simulink library "allActuatorPlant_cl"  (R2018b)
settings: Solver=VariableStepAuto  StartTime=0.0  StopTime=10.0  RelTol=1e-3
values from neighbouring files (symbols this model uses):
  unstretched_l = unstretched_l - ini_elongation - added_elongation    [ayazParams_init.m]    (also in multinode_wing_tail.m)
  X0 = cat(1,ini_Rcm_o,ini_O_Vcm_o,ini_euler_ang,ini_OwB,ini_platform_ang,ini_platform_vel,     ini_R1i_o,ini_R2i_o,ini_R3i_o,ini_O_V1i_o,ini_O_V2i_o,ini_O_V3i_o)    [ayazParams_init.m]    (also in multinode_wing_tail.m)
settings Model: Creator=mcobb  LastModifiedBy=embeato2

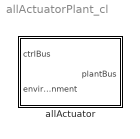
== system allActuatorPlant_cl ==
  allActuator : Subsystem

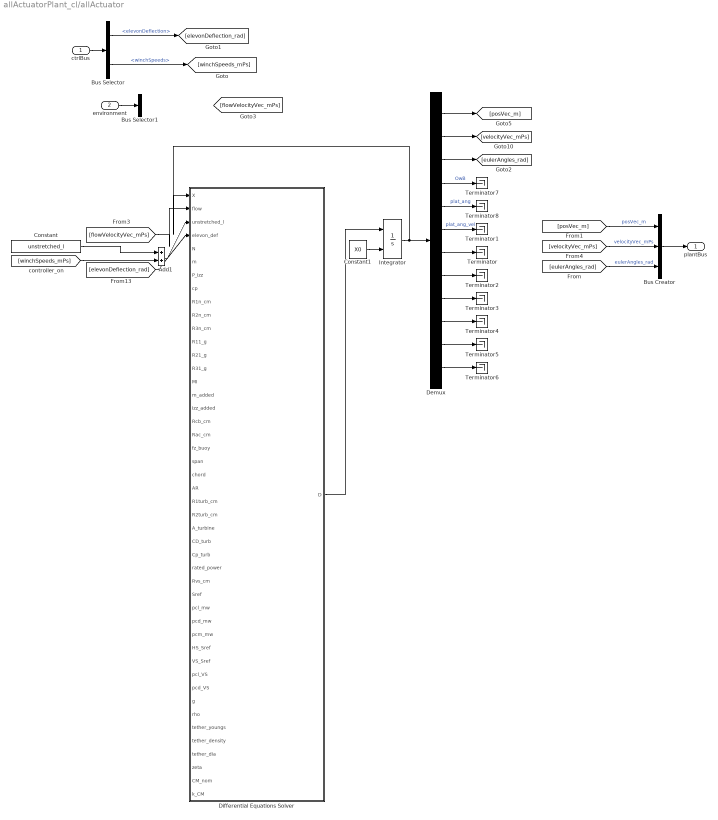
== system allActuatorPlant_cl/allActuator ==
  ctrlBus : Inport  OutDataTypeStr=Bus: ctrlBus
  environment : Inport  Port=2  OutDataTypeStr=Bus: envBus
  Add1 : Sum
  Bus Creator : BusCreator  Inputs=3  OutDataTypeStr=Bus: plantBus
  Bus Selector : BusSelector  OutputSignals=elevonDeflection,winchSpeeds
  Bus Selector1 : BusSelector  OutputSignals=windSpeed,windDir
  Constant : Constant  Value=unstretched_l
  Constant1 : Constant  Value=X0
  Demux : Demux  Outputs=[3,3,3,3,1,1,-1,-1,-1,-1,-1,-1]
  Differential Equations Solver : MATLAB Function  TreatAsAtomicUnit=on
  Integrator : Integrator  InitialConditionSource=external  InitialCondition=X0
  Terminator{,1..8} (9 alike) : Terminator
  plantBus : Outport  OutDataTypeStr=Bus: plantBus
  wires:
  Demux/3 -> [eulerAngles_rad]
  Integrator/1 -> Differential Equations Solver/1(X), Demux/1
  Demux/6 -> Terminator1/1  "plat_ang_vel"
  Constant/1 -> Add1/1
  Demux/7 -> Terminator/1
  Add1/1 -> Differential Equations Solver/3(unstretched_l)
  Differential Equations Solver/1(D) -> Integrator/1
  Demux/10 -> Terminator4/1
  Demux/4 -> Terminator7/1  "OwB"
  Demux/11 -> Terminator5/1
  Demux/12 -> Terminator6/1
  Demux/9 -> Terminator3/1
  Demux/1 -> [posVec_m]
  Demux/8 -> Terminator2/1
  [winchSpeeds_mPs] -> Add1/2
  Demux/5 -> Terminator8/1  "plat_ang"
  [elevonDeflection_rad] -> Differential Equations Solver/4(elevon_def)
  Demux/2 -> [velocityVec_mPs]
  [eulerAngles_rad] -> Bus Creator/3  "eulerAngles_rad"
  [posVec_m] -> Bus Creator/1  "posVec_m"
  Bus Creator/1 -> plantBus/1
  [flowVelocityVec_mPs] -> Differential Equations Solver/2(flow)
  Constant1/1 -> Integrator/2
  [velocityVec_mPs] -> Bus Creator/2  "velocityVec_mPs"
  ctrlBus/1 -> Bus Selector/1
  Bus Selector/1 -> [elevonDeflection_rad]  "<elevonDeflection>"
  Bus Selector/2 -> [winchSpeeds_mPs]  "<winchSpeeds>"
  environment/1 -> Bus Selector1/1

== matlab function allActuatorPlant_cl/allActuator/Differential Equations Solver ==
  data: X input; D output; flow input; unstretched_l input; elevon_def input; N input; m input; P_Izz input; cp input; R1n_cm input; R2n_cm input; R3n_cm input; R11_g input; R21_g input; R31_g input; MI input; m_added input; Izz_added input; Rcb_cm input; Rac_cm input; fz_buoy input; span input; chord input; AR input; R1turb_cm input; R2turb_cm input; A_turbine input; CD_turb input; Cp_turb input; rated_power input; Rvs_cm input; Sref input; pcl_mw input; pcd_mw input; pcm_mw input; HS_Sref input; VS_Sref input; pcl_VS input; pcd_VS input; g input; rho input; CD_cylinder parameter; tether_youngs input; tether_density input; tether_dia input; zeta input; CM_nom input; k_CM input
function D = multimode_ode(X,flow,unstretched_l,elevon_def, N, m, P_Izz, cp, R1n_cm, R2n_cm, ...
    R3n_cm, R11_g, R21_g, R31_g, MI, m_added, Izz_added, Rcb_cm, Rac_cm, fz_buoy, span, chord, AR, ...
    R1turb_cm, R2turb_cm, A_turbine, CD_turb, Cp_turb, rated_power, Rvs_cm, Sref, pcl_mw, pcd_mw, ...
    pcm_mw, HS_Sref, VS_Sref, pcl_VS, pcd_VS, g, rho, CD_cylinder, tether_youngs, tether_density, ...
    tether_dia, zeta, CM_nom, k_CM)

D = zeros(size(X));

% loader = load('sim_param.mat');
% 
% sim_param = loader.sim_param;

%% number of nodes
%N = sim_param.N;

% extract other values
%mass = sim_param.geom_param.mass;
%MI = sim_param.geom_param.MI;

%P_Izz = sim_param.platform_param.platform_Izz;
%cp = sim_param.platform_param.platform_damping;

%R1n_cm = sim_param.tether_imp_nodes.R1n_cm;
%R2n_cm = sim_param.tether_imp_nodes.R2n_cm;
%R3n_cm = sim_param.tether_imp_nodes.R3n_cm;

%R11_g = sim_param.tether_imp_nodes.R11_g;
%R21_g = sim_param.tether_imp_nodes.R21_g;
%R31_g = sim_param.tether_imp_nodes.R31_g;


%% constants
%m = mass;
Ixx = MI(1,1);
Iyy = MI(2,2);
Izz = MI(3,3);

%m_added = sim_param.geom_param.m_added;
%Izz_added = sim_param.geom_param.Izz_added;

%% extract values from state space
% lifting body values
Rcm_o = X(1:3,1);
O_Vcm_o = X(4:6,1);

euler_ang = X(7:9,1);
ph = euler_ang(1);
th = euler_ang(2);
ps = euler_ang(3);

% rotations
[oCb,bCo] = rotation_sequence(euler_ang);

OwB = X(10:12,1);
wx = OwB(1);
wy = OwB(2);
wz = OwB(3);

psi_p = X(13,1);
platform_ang_vel = X(14,1);

pCo = [cos(psi_p) sin(psi_p) 0; -sin(psi_p) cos(psi_p) 0; 0 0 1];
oCp = pCo';


% tether position and velocity components
R1i_o = X(15:(14 + 3*N),1);
R2i_o = X((15 + 3*N):(14 + 6*N),1);
R3i_o = X((15 + 6*N):(14 + 9*N),1);

O_V1i_o = X((15 + 9*N):(14 + 12*N),1);
O_V2i_o = X((15 + 12*N):(14 + 15*N),1);
O_V3i_o = X((15 + 15*N):(14 + 18*N),1);


%%  center of mass first derivatives
D(1:3,1) = O_Vcm_o;
D(7,1) = wx + sin(ph)*tan(th)*wy + cos(ph)*tan(th)*wz;
D(8,1) = cos(ph)*wy - sin(ph)*wz;
D(9,1) = sec(th)*sin(ph)*wy + cos(ph)*sec(th)*wz;

%% platofrm angle first derivates
D(13,1) = platform_ang_vel;
OwP = [0;0;platform_ang_vel];

%% grnd station first derivative
D(15:17,1) = [0;0;0];

%% changing first node first deivative
O_V1i_o(1:3,1) = oCp*(cross(OwP,R11_g));
O_V2i_o(1:3,1) = oCp*(cross(OwP,R21_g));
O_V3i_o(1:3,1) = oCp*(cross(OwP,R31_g));

%% changing last node first deivative
O_V1i_o((end-2):end,1) = O_Vcm_o + oCb*(cross(OwB,R1n_cm));
O_V2i_o((end-2):end,1)=  O_Vcm_o + oCb*(cross(OwB,R2n_cm));
O_V3i_o((end-2):end,1)=  O_Vcm_o + oCb*(cross(OwB,R3n_cm));

%% tether nodes first derivatives
D(15:(14 + 3*N),1) = O_V1i_o;
D((15 + 3*N):(14 + 6*N),1) = O_V2i_o;
D((15 + 6*N):(14 + 9*N),1) = O_V3i_o;

%% DEFINE SIM_PARAM

sim_param.N = N;

sim_param.geom_param.mass = m;
sim_param.geom_param.center_of_buoy = Rcb_cm;
sim_param.geom_param.aero_center = Rac_cm;
sim_param.geom_param.F_buoy = fz_buoy;
sim_param.geom_param.span = span;
sim_param.geom_param.chord = chord;
sim_param.geom_param.AR = AR;

sim_param.turbine_param.R1turb_cm = R1turb_cm;
sim_param.turbine_param.R2turb_cm = R2turb_cm;
sim_param.turbine_param.A_turbine = A_turbine;
sim_param.turbine_param.CD_turb = CD_turb;
sim_param.turbine_param.Cp_turb = Cp_turb;
sim_param.turbine_param.rated_power = rated_power;

sim_param.aero_param.Rvs_cm = Rvs_cm;
sim_param.aero_param.Sref = Sref;
sim_param.aero_param.pcl_mw = pcl_mw;
sim_param.aero_param.pcd_mw = pcd_mw;
sim_param.aero_param.pcm_mw = pcm_mw;
sim_param.aero_param.HS_Sref = HS_Sref;
sim_param.aero_param.VS_Sref = VS_Sref;
sim_param.aero_param.pcl_VS = pcl_VS;
sim_param.aero_param.pcd_VS = pcd_VS;

sim_param.tether_imp_nodes.R1n_cm = R1n_cm;
sim_param.tether_imp_nodes.R2n_cm = R2n_cm;
sim_param.tether_imp_nodes.R3n_cm = R3n_cm;
sim_param.tether_imp_nodes.R11_g = R11_g;
sim_param.tether_imp_nodes.R21_g = R21_g;
sim_param.tether_imp_nodes.R31_g = R31_g;


sim_param.env_param.grav = g;
sim_param.env_param.density = rho;

sim_param.tether_param.CD_cylinder = CD_cylinder;
sim_param.tether_param.tether_youngs = tether_youngs;
sim_param.tether_param.tether_density = tether_density;
sim_param.tether_param.tether_diameter = tether_dia;
sim_param.tether_param.damping_ratio = zeta;

sim_param.elevons_param.CM_nom = CM_nom;
sim_param.elevons_param.k_CM = k_CM;


%% EXTERNAL FORCES AND TORQUES
op = multinode_F_and_T_external(sim_param,flow,unstretched_l,elevon_def,Rcm_o,R1i_o,R2i_o,R3i_o,...
    O_Vcm_o,O_V1i_o,O_V2i_o,O_V3i_o,OwB,euler_ang,psi_p);

O_F_ext = op.O_F_ext;
B_T_ext = op.B_T_ext;
sum_1_f = op.sum_1_f;
sum_2_f = op.sum_2_f;
sum_3_f = op.sum_3_f;
T_o_ext = op.T_o_ext;

Tx = B_T_ext(1);
Ty = B_T_ext(2);
Tz = B_T_ext(3);

% mass at each node
tether_masses = op.tether_masses;

m1i = tether_masses(1)/N;
m2i = tether_masses(2)/N;
m3i = tether_masses(3)/N;

%% center of mass second derivatives
% added mass
mass_matrix = [1/(m+m_added(1)) 0 0;0 1/(m+m_added(2)) 0;0 0 1/(m+m_added(3))];

D(4:6,1) = oCb*(mass_matrix*(bCo*O_F_ext));
D(10,1) = (1/Ixx)*(Tx + (Iyy - Izz)*wy*wz);
D(11,1) = (1/Iyy)*(Ty + (Izz - Ixx)*wx*wz);
D(12,1) = (1/(Izz+Izz_added))*(Tz + (Ixx - Iyy)*wx*wy);

OaB = D(10:12,1);

%% platform angle second derivative
D(14,1) = (T_o_ext/P_Izz) - cp*platform_ang_vel;
OaP = [0;0;D(14,1)];

%% tether nodes 2nd derivatives

for i = 1:N
    
    if i == 1
        D((14 + 9*N + 3*i - 2):(14 + 9*N + 3*i),1) = oCp*( cross(OaP,R11_g) +  cross(OwP,(cross(OwP,R11_g))) );
        D((14 + 12*N + 3*i - 2):(14 + 12*N + 3*i),1) = oCp*( cross(OaP,R21_g) +  cross(OwP,(cross(OwP,R21_g))) );
        D((14 + 15*N + 3*i - 2):(14 + 15*N + 3*i),1) = oCp*( cross(OaP,R31_g) +  cross(OwP,(cross(OwP,R31_g))) );
        
    elseif i>1 && i<N
        
        D((14 + 9*N + 3*i - 2):(14 + 9*N + 3*i),1) = (1/m1i)*sum_1_f(:,i);
        D((14 + 12*N + 3*i - 2):(14 + 12*N + 3*i),1) = (1/m2i)*sum_2_f(:,i);
        D((14 + 15*N + 3*i - 2):(14 + 15*N + 3*i),1) = (1/m3i)*sum_3_f(:,i);
        
    elseif i == N
        
        D((14 + 9*N + 3*i - 2):(14 + 9*N + 3*i),1) = D(4:6,1) + ...
            oCb*( cross(OaB,R1n_cm) +  cross(OwB,(cross(OwB,R1n_cm))) );
        
        
        D((14 + 12*N + 3*i - 2):(14 + 12*N + 3*i),1) =  D(4:6,1) + ...
            oCb*( cross(OaB,R2n_cm) +  cross(OwB,(cross(OwB,R2n_cm))) ) ;
        
        D((14 + 15*N + 3*i - 2):(14 + 15*N + 3*i),1) =  D(4:6,1) + ...
            oCb*( cross(OaB,R3n_cm) +  cross(OwB,(cross(OwB,R3n_cm))) );
        
    end
    
    
end


end
